simulink model "sm_tVtest_belt_IdlerArm_i2u0r3_lowerframe"  (R2026a)
settings: Solver=ode23t  StopTime=16  AbsTol=1e-3  EnableMultiTasking=on
StartFcn:
  | tic
StopFcn:
  | Elapsed_Sim_Time = toc;
  | disp(['Elapsed Sim Time = ' num2str(Elapsed_Sim_Time)]);
undefined symbols (not defined in the file or in its folder): A, L1, L2, L3, qSegSpr_seg45i2u0r3, S, sprk_pitch_rad, X, Y, Z
libraries: sm_lib x7, sm_trackV_lib_belt_contact_internal_sets x7, fl_lib x2, nesl_utility x2, sm_trackV_lib_chain_underc_elem x1, simulink x1, sm_trackV_lib_terrain_contact_s45 x1, sm_trackV_lib_belt_track_s45 x1, sm_trackV_lib_belt_underc_idlerArm_i2u0l3 x1
Description:
  | Belt with Undercarriage, Ground Contact Point Cloud
  | Copyright 2024-2026 The MathWorks, Inc.
settings Model: Creator=smiller  LastModifiedBy=smiller
settings DataIOCC: SignalLoggingName=logsout_sm_tVtest_belt_IdlerArm_i2u0r3_lowerframe
settings DebuggingCC: SubsystemReferenceDiagnosticForUnitTest=warning
settings SimscapeCC: SimscapeNominalValues="[{\"value\":\"1\",\"unit\":\"A\"},{\"value\":\"1\",\"unit\":\"bar\"},{\"value\":\"1\",\"unit\":\"cm^2\"},{\"value\":\"1\",\"unit\":\"cm^3/s\"},{\"value\":\"1\",\"unit\":\"kJ/kg\"},{\"value\":\"1\",\"unit\":\"kW\"},{\"value\":\"1\",\"unit\":\"l\"},{\"value\":\"1\",\"unit\":\"N\"},{\"value\":\"1\",\"unit\":\"N*m\"},{\"value\":\"1\",\"unit\":\"V\"}]"  SimscapeLogSimulationStatistics=on  SimscapeLogName=simlog_sm_tVtest_belt_IdlerArm_i2u0r3_lowerframe  SimscapeLogLimitData=off
settings DiagnosticsConfigSet: SimMechanicsUnconnectedFramePorts=none
settings ExplorerConfigSet: InternalSimMechanicsExplorerSettings="<ExplorerConfiguration><canonicalview>default</canonicalview><AnimationSetting><BasePlaybackSpeed>1.0</BasePlaybackSpeed><PlaybackSpeedFactor>1.0</PlaybackSpeedFactor></AnimationSetting><TilePanel><TileInfo><Tiles Columns=\"1\" Count=\"1\" Rows=\"1\"><Column Weight=\"1\"/><Row Weight=\"1\"/><Tile Height=\"1\" Width=\"1\" X=\"0\" Y=\"0\"/></Tiles></TileInfo><SceneInfo><SceneViewer><BGColor><R>1</R><G>1</G><B>1</B></BGColor><Camera><DoPerspective>off</DoPerspective><Position><X>0.47068243127928272</X><Y>-1.75489189973030935</Y><Z>1.25342844941222076</Z></Position><Center><X>-0.0540333939973325975</X><Y>-0.199725656684764663</Y><Z>0.955761903192511197</Z></Center><Up><X>-0.029483751236791006</X><Y>0.178305307946765135</Y><Z>0.983533388132307618</Z></Up><ViewLimDist>1</ViewLimDist><YLim>1.28706962276995207</YLim><XLim>2.19495206711441337</XLim></Camera></SceneViewer></SceneInfo></TilePanel><MechEditorPanel><Cameras/><GfxPanelCameraMap/><VideoCreator><PlaybackSpeedRatio>1.0</PlaybackSpeedRatio><FrameRate>30</FrameRate><VideoFormat>Motion JPEG AVI</VideoFormat><FrameSize>auto</FrameSize></VideoCreator></MechEditorPanel></ExplorerConfiguration>"

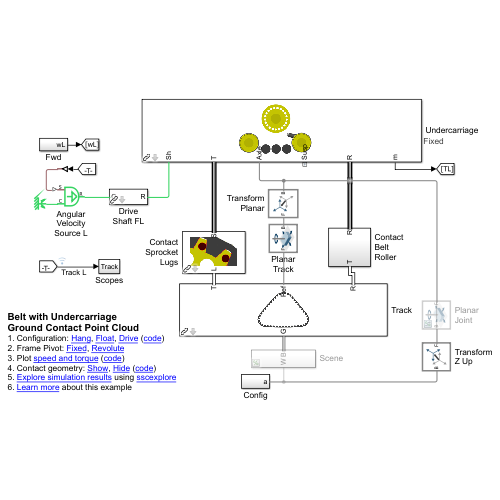
[thumbnail: Simulink's stored preview of the top-level diagram]
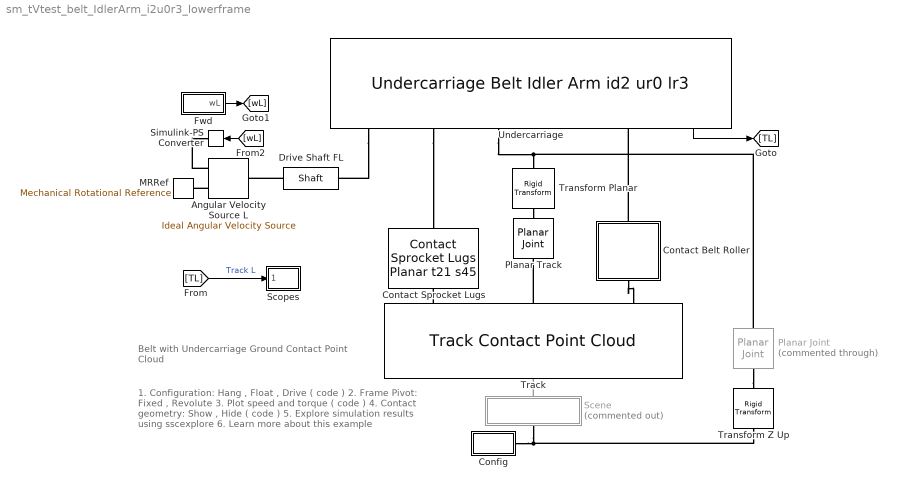
== system sm_tVtest_belt_IdlerArm_i2u0r3_lowerframe ==
  note: Belt with Undercarriage
      | Ground Contact Point Cloud
  note: 1. Configuration: Hang , Float , Drive ( code )
      | 2. Frame Pivot: Fixed , Revolute
      | 3. Plot speed and torque ( code )
      | 4. Contact geometry: Show , Hide ( code )
      | 5. Explore simulation results using sscexplore
      | 6. Learn more about this example
  Angular Velocity Source L : fl_lib/Mechanical/Mechanical Sources/Ideal Angular Velocity Source
  Config : Subsystem
  Contact Belt Roller : Subsystem
  Contact Sprocket Lugs : sm_trackV_lib_belt_contact_internal_sets/Contact Sprocket Lugs Planar t21 s45  K_SprocketLug=Trac.Contact.SprocketLug.K  B_SprocketLug=Trac.Contact.SprocketLug.B  TW_SprocketLug=Trac.Contact.SprocketLug.TW
  Drive Shaft FL : sm_trackV_lib_chain_underc_elem/Shaft  k_shaft=Excv.Drive.Shaft.k  b_shaft=Excv.Drive.Shaft.b
  Fwd : Subsystem  VariantControl=Fwd
  MRRef : fl_lib/Mechanical/Rotational Elements/Mechanical Rotational Reference
  Planar Joint : sm_lib/Joints/Planar Joint  Commented=through  JointMode=Normal  CompositeWrenchDir=FollowerOnBase  CompositeWrenchFrame=BaseFrame  SenseConstraintForce=off  SenseConstraintTorque=off  SenseTotalForce=off  SenseTotalTorque=off  PxPositionTargetSpecify=off  PxPositionTargetPriority=High  PxPositionTargetValue=0  PxPositionTargetValueUnits=m  PxVelocityTargetSpecify=off  PxVelocityTargetPriority=High  PxVelocityTargetValue=0  PxVelocityTargetValueUnits=m/s  PxEquilibriumPosition=0  PxEquilibriumPositionUnits=m  PxSpringStiffness=0  PxSpringStiffnessUnits=N/m  PxDampingCoefficient=0  PxDampingCoefficientUnits=N/(m/s)  PxLowerLimitSpecify=off  PxLowerLimitBound=-1  PxLowerLimitBoundUnits=m  PxLowerLimitStiffness=1e6  PxLowerLimitStiffnessUnits=N/m  PxLowerLimitDamping=1e3  PxLowerLimitDampingUnits=N/(m/s)  PxLowerLimitTransitionRegionWidth=1e-4  PxLowerLimitTransitionRegionWidthUnits=m  PxUpperLimitSpecify=off  PxUpperLimitBound=1  PxUpperLimitBoundUnits=m  PxUpperLimitStiffness=1e6  PxUpperLimitStiffnessUnits=N/m  PxUpperLimitDamping=1e3  PxUpperLimitDampingUnits=N/(m/s)  PxUpperLimitTransitionRegionWidth=1e-4  PxUpperLimitTransitionRegionWidthUnits=m  PxTorqueActuationMode=NoTorque  PxMotionActuationMode=ComputedMotion  PxSensePosition=off  PxSenseVelocity=off  PxSenseAcceleration=off  PxSenseTorqueForce=off  PxSenseLowerLimitTorqueForce=off  PxSenseUpperLimitTorqueForce=off  PyPositionTargetSpecify=off  PyPositionTargetPriority=High  PyPositionTargetValue=0  PyPositionTargetValueUnits=m  PyVelocityTargetSpecify=off  PyVelocityTargetPriority=High  PyVelocityTargetValue=0  PyVelocityTargetValueUnits=m/s  PyEquilibriumPosition=0  PyEquilibriumPositionUnits=m  PySpringStiffness=0  PySpringStiffnessUnits=N/m  PyDampingCoefficient=0  PyDampingCoefficientUnits=N/(m/s)  PyLowerLimitSpecify=off  PyLowerLimitBound=-1  PyLowerLimitBoundUnits=m  PyLowerLimitStiffness=1e6  PyLowerLimitStiffnessUnits=N/m  PyLowerLimitDamping=1e3  PyLowerLimitDampingUnits=N/(m/s)  PyLowerLimitTransitionRegionWidth=1e-4  PyLowerLimitTransitionRegionWidthUnits=m  PyUpperLimitSpecify=off  PyUpperLimitBound=1  PyUpperLimitBoundUnits=m  PyUpperLimitStiffness=1e6  PyUpperLimitStiffnessUnits=N/m  PyUpperLimitDamping=1e3  PyUpperLimitDampingUnits=N/(m/s)  PyUpperLimitTransitionRegionWidth=1e-4  PyUpperLimitTransitionRegionWidthUnits=m  PyTorqueActuationMode=NoTorque  PyMotionActuationMode=ComputedMotion  PySensePosition=off  PySenseVelocity=off  PySenseAcceleration=off  PySenseTorqueForce=off  PySenseLowerLimitTorqueForce=off  PySenseUpperLimitTorqueForce=off  RzPositionTargetSpecify=off  RzPositionTargetPriority=High  RzPositionTargetValue=0  RzPositionTargetValueUnits=deg  RzVelocityTargetSpecify=off  RzVelocityTargetPriority=High  RzVelocityTargetValue=0  RzVelocityTargetValueUnits=deg/s  RzEquilibriumPosition=0  RzEquilibriumPositionUnits=deg  RzSpringStiffness=0  RzSpringStiffnessUnits=N*m/deg  RzDampingCoefficient=0  RzDampingCoefficientUnits=N*m/(deg/s)  RzLowerLimitSpecify=off  RzLowerLimitBound=-90  RzLowerLimitBoundUnits=deg  RzLowerLimitStiffness=1e4  RzLowerLimitStiffnessUnits=N*m/deg  RzLowerLimitDamping=10  RzLowerLimitDampingUnits=N*m/(deg/s)  RzLowerLimitTransitionRegionWidth=0.1  RzLowerLimitTransitionRegionWidthUnits=deg  RzUpperLimitSpecify=off  RzUpperLimitBound=90  RzUpperLimitBoundUnits=deg  RzUpperLimitStiffness=1e4  RzUpperLimitStiffnessUnits=N*m/deg  RzUpperLimitDamping=10  RzUpperLimitDampingUnits=N*m/(deg/s)  RzUpperLimitTransitionRegionWidth=0.1  RzUpperLimitTransitionRegionWidthUnits=deg  RzTorqueActuationMode=NoTorque  RzMotionActuationMode=ComputedMotion  RzSensePosition=off  RzSenseVelocity=off  RzSenseAcceleration=off  RzSenseTorqueForce=off  RzSenseLowerLimitTorqueForce=off  RzSenseUpperLimitTorqueForce=off
  Planar Track : sm_lib/Joints/Planar Joint  JointMode=Normal  CompositeWrenchDir=FollowerOnBase  CompositeWrenchFrame=BaseFrame  SenseConstraintForce=off  SenseConstraintTorque=off  SenseTotalForce=off  SenseTotalTorque=off  PxPositionTargetSpecify=off  PxPositionTargetPriority=High  PxPositionTargetValue=0  PxPositionTargetValueUnits=m  PxVelocityTargetSpecify=off  PxVelocityTargetPriority=High  PxVelocityTargetValue=0  PxVelocityTargetValueUnits=m/s  PxEquilibriumPosition=0  PxEquilibriumPositionUnits=m  PxSpringStiffness=0  PxSpringStiffnessUnits=N/m  PxDampingCoefficient=0  PxDampingCoefficientUnits=N/(m/s)  PxLowerLimitSpecify=off  PxLowerLimitBound=-1  PxLowerLimitBoundUnits=m  PxLowerLimitStiffness=1e6  PxLowerLimitStiffnessUnits=N/m  PxLowerLimitDamping=1e3  PxLowerLimitDampingUnits=N/(m/s)  PxLowerLimitTransitionRegionWidth=1e-4  PxLowerLimitTransitionRegionWidthUnits=m  PxUpperLimitSpecify=off  PxUpperLimitBound=1  PxUpperLimitBoundUnits=m  PxUpperLimitStiffness=1e6  PxUpperLimitStiffnessUnits=N/m  PxUpperLimitDamping=1e3  PxUpperLimitDampingUnits=N/(m/s)  PxUpperLimitTransitionRegionWidth=1e-4  PxUpperLimitTransitionRegionWidthUnits=m  PxTorqueActuationMode=NoTorque  PxMotionActuationMode=ComputedMotion  PxSensePosition=off  PxSenseVelocity=off  PxSenseAcceleration=off  PxSenseTorqueForce=off  PxSenseLowerLimitTorqueForce=off  PxSenseUpperLimitTorqueForce=off  PyPositionTargetSpecify=off  PyPositionTargetPriority=Low  PyPositionTargetValue=-sprk_pitch_rad  PyPositionTargetValueUnits=m  PyVelocityTargetSpecify=off  PyVelocityTargetPriority=High  PyVelocityTargetValue=0  PyVelocityTargetValueUnits=m/s  PyEquilibriumPosition=0  PyEquilibriumPositionUnits=m  PySpringStiffness=0  PySpringStiffnessUnits=N/m  PyDampingCoefficient=0  PyDampingCoefficientUnits=N/(m/s)  PyLowerLimitSpecify=off  PyLowerLimitBound=-1  PyLowerLimitBoundUnits=m  PyLowerLimitStiffness=1e6  PyLowerLimitStiffnessUnits=N/m  PyLowerLimitDamping=1e3  PyLowerLimitDampingUnits=N/(m/s)  PyLowerLimitTransitionRegionWidth=1e-4  PyLowerLimitTransitionRegionWidthUnits=m  PyUpperLimitSpecify=off  PyUpperLimitBound=1  PyUpperLimitBoundUnits=m  PyUpperLimitStiffness=1e6  PyUpperLimitStiffnessUnits=N/m  PyUpperLimitDamping=1e3  PyUpperLimitDampingUnits=N/(m/s)  PyUpperLimitTransitionRegionWidth=1e-4  PyUpperLimitTransitionRegionWidthUnits=m  PyTorqueActuationMode=NoTorque  PyMotionActuationMode=ComputedMotion  PySensePosition=off  PySenseVelocity=off  PySenseAcceleration=off  PySenseTorqueForce=off  PySenseLowerLimitTorqueForce=off  PySenseUpperLimitTorqueForce=off  RzPositionTargetSpecify=on  RzPositionTargetPriority=High  RzPositionTargetValue=0  RzPositionTargetValueUnits=deg  RzVelocityTargetSpecify=off  RzVelocityTargetPriority=High  RzVelocityTargetValue=0  RzVelocityTargetValueUnits=deg/s  RzEquilibriumPosition=0  RzEquilibriumPositionUnits=deg  RzSpringStiffness=0  RzSpringStiffnessUnits=N*m/deg  RzDampingCoefficient=0  RzDampingCoefficientUnits=N*m/(deg/s)  RzLowerLimitSpecify=off  RzLowerLimitBound=-90  RzLowerLimitBoundUnits=deg  RzLowerLimitStiffness=1e4  RzLowerLimitStiffnessUnits=N*m/deg  RzLowerLimitDamping=10  RzLowerLimitDampingUnits=N*m/(deg/s)  RzLowerLimitTransitionRegionWidth=0.1  RzLowerLimitTransitionRegionWidthUnits=deg  RzUpperLimitSpecify=off  RzUpperLimitBound=90  RzUpperLimitBoundUnits=deg  RzUpperLimitStiffness=1e4  RzUpperLimitStiffnessUnits=N*m/deg  RzUpperLimitDamping=10  RzUpperLimitDampingUnits=N*m/(deg/s)  RzUpperLimitTransitionRegionWidth=0.1  RzUpperLimitTransitionRegionWidthUnits=deg  RzTorqueActuationMode=NoTorque  RzMotionActuationMode=ComputedMotion  RzSensePosition=off  RzSenseVelocity=off  RzSenseAcceleration=off  RzSenseTorqueForce=off  RzSenseLowerLimitTorqueForce=off  RzSenseUpperLimitTorqueForce=off
  Scene : Subsystem  Commented=on
  Scopes : Subsystem
  Simulink-PS Converter : nesl_utility/Simulink-PS Converter  PhysicalDomain=network_engine_domain  SubClassName=ps_input  LeftPortType=input  RightPortType=output  PseudoPeriodic=off  Frequencies=[]  NoiseDistribution=none  NoiseParameters=[]  Unit=1  AffineConversion=off  FilteringAndDerivatives=provide  SimscapeFilterOrder=1  InputFilterTimeConstant=0.001  UdotUserProvided=0
  Track : sm_trackV_lib_belt_track_s45/Track Contact Point Cloud  carc_len=Trac.Belt.l  carc_wid=Trac.Belt.w  carc_thk=Trac.Belt.pad_h  carc_mass=Trac.Belt.mass  carc_cg=Trac.Belt.cg  carc_moi=Trac.Belt.moi  carc_poi=Trac.Belt.poi  carc_clr=Trac.Belt.clr  carc_opc=Trac.Belt.opc  lug_hei=Trac.Belt.Lug.h  lug_lb=Trac.Belt.Lug.lb  lug_lt=Trac.Belt.Lug.lt  lug_w=Trac.Belt.Lug.w  lug_xc=Trac.Belt.Lug.xc  lug_clr=Trac.Belt.clr  lug_opc=Trac.Belt.opc  jointTargets=track_seg_tgts_seg45i2u0r3  trackDamping=Trac.Belt.damping  lug_line_clr=Trac.Belt.lug_contact.clr  lug_line_opc=Trac.Belt.lug_contact.opc  carc_line_clr=Trac.Belt.carcass_contact.clr  carc_line_opc=Trac.Belt.carcass_contact.opc  ptcld_belt=Trac.Belt.ground_contact.ptcld.pts  ptcld_belt_rad=Trac.Belt.ground_contact.ptcld.rad  ptcld_belt_clr=Trac.Belt.ground_contact.ptcld.clr  ptcld_belt_opc=Trac.Belt.ground_contact.ptcld.opc
  Transform Planar : sm_lib/Frames and Transforms/Rigid Transform  RotationMethod=StandardAxis  FollAlignAxisA=+X  BaseAlignAxisA=+Y  FollAlignAxisB=+Y  BaseAlignAxisB=+Z  RotationStandardAxis=+Z  RotationAngle=-qSegSpr_seg45i2u0r3/2  RotationAngleUnits=deg  RotationArbitraryAxis=[0 0 1]  RotationSequenceAxes=FollowerAxes  RotationSequence=XYX  RotationSequenceAngles=[0 0 0]  RotationSequenceAnglesUnits=deg  RotationMatrix=[1 0 0; 0 1 0; 0 0 1]  Quaternion=[1 0 0 0]  TranslationMethod=StandardAxis  TranslationCartesianOffset=[0 0 0]  TranslationCartesianOffsetUnits=m  TranslationStandardAxis=+Y  TranslationStandardOffset=-sprk_pitch_rad  TranslationStandardOffsetUnits=m  TranslationROffset=0  TranslationROffsetUnits=m  TranslationThetaOffset=0  TranslationThetaOffsetUnits=deg  TranslationZOffset=0  TranslationZOffsetUnits=m
  Transform Z Up : sm_lib/Frames and Transforms/Rigid Transform  RotationMethod=StandardAxis  FollAlignAxisA=+X  BaseAlignAxisA=+Y  FollAlignAxisB=+Y  BaseAlignAxisB=+Z  RotationStandardAxis=+X  RotationAngle=-90  RotationAngleUnits=deg  RotationArbitraryAxis=[0 0 1]  RotationSequenceAxes=FollowerAxes  RotationSequence=XYX  RotationSequenceAngles=[0 0 0]  RotationSequenceAnglesUnits=deg  RotationMatrix=[1 0 0; 0 1 0; 0 0 1]  Quaternion=[1 0 0 0]  TranslationMethod=StandardAxis  TranslationCartesianOffset=[0 0 0]  TranslationCartesianOffsetUnits=m  TranslationStandardAxis=+Z  TranslationStandardOffset=1.5  TranslationStandardOffsetUnits=m  TranslationROffset=0  TranslationROffsetUnits=m  TranslationThetaOffset=0  TranslationThetaOffsetUnits=deg  TranslationZOffset=0  TranslationZOffsetUnits=m
  Undercarriage : sm_trackV_lib_belt_underc_idlerArm_i2u0l3/Undercarriage Belt Idler Arm id2 ur0 lr3  popup_leftOrRight=Right  sprk_rad_roll=Trac.Sprocket.Roller.rad  sprk_wid_roll=Trac.Sprocket.Roller.wid  sprk_clr=Trac.Sprocket.Roller.clr  sprk_opc=Trac.Sprocket.Roller.opc  sprk_rim_ir=Trac.Sprocket.Rim.rad_inner  sprk_rim_thk=Trac.Sprocket.Rim.thk  sprk_rim_spoke_xc=Trac.Sprocket.Rim.spoke_xc  sprk_rad_pitch=Trac.Sprocket.Spoke.pitch_rad  sprk_spoke_rad=Trac.Sprocket.Spoke.rad  sprk_spoke_len=Trac.Sprocket.Spoke.len  sprk_spoke_num=Trac.Sprocket.nSpokes  sprk_contgeo_roller_clr=Trac.Sprocket.roller_contact.clr  sprk_contgeo_roller_opc=Trac.Sprocket.roller_contact.opc  sprk_contgeo_spoke_clr=Trac.Sprocket.spoke_contact.clr  sprk_contgeo_spoke_opc=Trac.Sprocket.spoke_contact.opc  idlerR_rad=Trac.IdlerR.rad  idlerF_rad=Trac.IdlerF.rad  idlerR_len=Trac.IdlerR.len  idlerF_len=Trac.IdlerF.len  idlerR_rho=Trac.IdlerR.rho  idlerF_rho=Trac.IdlerF.rho  idlerR_wheel_clr=Trac.IdlerR.Wheel.clr  idlerF_wheel_clr=Trac.IdlerF.Wheel.clr  idlerR_rim_rad=Trac.IdlerR.Rim.rad  idlerF_rim_rad=Trac.IdlerF.Rim.rad  idlerR_rim_hub_rad=Trac.IdlerR.Rim.hub_rad  idlerF_rim_hub_rad=Trac.IdlerF.Rim.hub_rad  idlerR_rim_xc=Trac.IdlerR.Rim.rim_xc  idlerF_rim_xc=Trac.IdlerF.Rim.rim_xc  idlerR_clr=Trac.IdlerR.clr  idlerF_clr=Trac.IdlerF.clr  idlerR_opc=Trac.IdlerR.opc  idlerF_opc=Trac.IdlerF.opc  idlerR_axle_rad=Trac.IdlerR.Axle.rad  idlerF_axle_rad=Trac.IdlerF.Axle.rad  idlerR_axle_len=Trac.IdlerR.Axle.len  idlerF_axle_len=Trac.IdlerF.Axle.len  idlerR_axle_rho=Trac.IdlerR.Axle.rho  idlerF_axle_rho=Trac.IdlerF.Axle.rho  idlerR_axle_clr=Trac.IdlerR.Axle.clr  idlerF_axle_clr=Trac.IdlerF.Axle.clr  idlerR_axle_opc=Trac.IdlerR.Axle.opc  idlerF_axle_opc=Trac.IdlerF.Axle.opc  idlerR_contgeo_clr=Trac.IdlerR.belt_contact.clr  idlerF_contgeo_clr=Trac.IdlerF.belt_contact.clr  idlerR_contgeo_opc=Trac.IdlerR.belt_contact.opc  idlerF_contgeo_opc=Trac.IdlerF.belt_contact.opc  arm_idlerc=Trac.IdlerArm.Pivot_to_Idler  arm_tens_x=Trac.IdlerArm.Pivot_to_TensionerX  arm_tens_y=Trac.IdlerArm.Pivot_to_TensionerY  arm_wid=Trac.IdlerArm.wid  arm_thk=Trac.IdlerArm.thk  arm_rho=Trac.IdlerArm.rho  arm_clr=Trac.IdlerArm.clr  arm_opc=Trac.IdlerArm.opc  roller_lower_len=Trac.Roller.Lower.len  roller_lower_rad=Trac.Roller.Lower.rad  roller_lower_rho=Trac.Roller.Lower.rho  roller_lower_clr=Trac.Roller.Lower.clr  roller_lower_opc=Trac.Roller.Lower.opc  roller_lower_rim_thk=Trac.Roller.Lower.rim_thk  roller_lower_rim_len=Trac.Roller.Lower.rim_len  roller_lower_axle_len=Trac.Roller.Lower.Axle.len  roller_lower_axle_rad=Trac.Roller.Lower.Axle.rad  roller_lower_axle_rho=Trac.Roller.Lower.Axle.rho  roller_lower_axle_clr=Trac.Roller.Lower.Axle.clr  roller_lower_axle_opc=Trac.Roller.Lower.Axle.opc  roller_lower_contgeo_clr=Trac.Roller.Lower.belt_contact.clr  roller_lower_contgeo_opc=Trac.Roller.Lower.belt_contact.opc  tensioner_cyl_len=Trac.IdlerF.Tensioner.cyl.len  tensioner_cyl_rad=Trac.IdlerF.Tensioner.cyl.rad  tensioner_cyl_rho=Trac.IdlerF.Tensioner.cyl.rho  tensioner_cyl_clr=Trac.IdlerF.Tensioner.cyl.clr  tensioner_cyl_opc=Trac.IdlerF.Tensioner.cyl.opc  tensioner_pist_len=Trac.IdlerF.Tensioner.piston.len  tensioner_pist_rad=Trac.IdlerF.Tensioner.piston.rad  tensioner_pist_rho=Trac.IdlerF.Tensioner.piston.rho  tensioner_pist_clr=Trac.IdlerF.Tensioner.piston.clr  tensioner_pist_opc=Trac.IdlerF.Tensioner.piston.opc  tensioner_br_len=Trac.IdlerF.Tensioner.bracket.len  tensioner_br_width=Trac.IdlerF.Tensioner.bracket.wid  tensioner_br_height=Trac.IdlerF.Tensioner.bracket.height  tensioner_br_thk=Trac.IdlerF.Tensioner.bracket.thk  tensioner_br_rho=Trac.IdlerF.Tensioner.bracket.rho  tensioner_br_clr=Trac.IdlerF.Tensioner.bracket.clr  tensioner_br_opc=Trac.IdlerF.Tensioner.bracket.opc  tensioner_eqpos=Trac.IdlerF.Tensioner.xeq  tensioner_x0=Trac.IdlerF.Tensioner.x0  tensioner_k=Trac.IdlerF.Tensioner.K  tensioner_b=Trac.IdlerF.Tensioner.B  popup_trackFrame=Fixed  roller_lower_x=Trac.Frame.SprkOffLon.Lower  axle_x=Trac.Frame.SprkOffLon.Axle  idlerFix_x=Trac.Frame.SprkOffLon.IdlerR  frame_pivot_x=Trac.Frame.SprkOffLon.PivotFra  tensionC_x=Trac.Frame.SprkOffLon.TensionC  idlerArm_x=Trac.Frame.SprkOffLon.IdlerArm  roller_lower_y=Trac.Frame.SprkOffVer.Lower  axle_y=Trac.Frame.SprkOffVer.Axle  idlerArm_y=Trac.Frame.SprkOffVer.IdlerArm  idlerFix_y=Trac.Frame.SprkOffVer.IdlerR  frame_pivot_y=Trac.Frame.SprkOffVer.PivotFra  tensionC_y=Trac.Frame.SprkOffVer.TensionC  frame_cg_offset=Trac.Frame.TrackFrame.CG  frame_mass=Trac.Frame.TrackFrame.Mass  frame_moi=Trac.Frame.TrackFrame.MOI  frame_poi=Trac.Frame.TrackFrame.POI  frame_roller_cg_offset=Trac.Frame.SprkFrame.CG  frame_roller_mass=Trac.Frame.SprkFrame.Mass  frame_roller_moi=Trac.Frame.SprkFrame.MOI  frame_roller_poi=Trac.Frame.SprkFrame.POI  roller_frame_pivot_range=Trac.Frame.PivotFra.Range  roller_frame_pivot_k=Trac.Frame.PivotFra.LimitK  roller_frame_pivot_b=Trac.Frame.PivotFra.LimitB  roller_frame_pivot_tw=Trac.Frame.PivotFra.LimitTW  frame_susp_offset=Trac.Frame.SuspOffset  popup_sense_roller=Actuator Torque
      settings: AttributesFormatString=%<popup_trackFrame>
  wires:
  Fwd/1(wL) -> [wL]
  [wL] -> Simulink-PS Converter/1
  Undercarriage/1 -> [TL]
  [TL] -> Scopes/1(Track)  "Track L"
  connections:
  Transform Planar/RConn1 -- Planar Track/LConn1
  Angular Velocity Source L/RConn2 -- MRRef/LConn1
  Drive Shaft FL/LConn1 -- Angular Velocity Source L/LConn1
  Undercarriage/RConn5 -- Drive Shaft FL/RConn1
  Contact Belt Roller/LConn1 -- Track/RConn3
  Contact Belt Roller/RConn1 -- Undercarriage/RConn1
  Track/RConn2 -- Planar Track/RConn1
  Track/RConn1 -- Contact Sprocket Lugs/RConn1
  Undercarriage/RConn4 -- Contact Sprocket Lugs/LConn1
  Planar Joint/RConn1 -- Transform Planar/LConn1 -- Undercarriage/RConn3
  Planar Joint/LConn1 -- Transform Z Up/RConn1
  Angular Velocity Source L/RConn1 -- Simulink-PS Converter/RConn1
  Transform Z Up/LConn1 -- Config/RConn1 -- Scene/LConn1
  Scene/RConn1 -- Track/LConn1

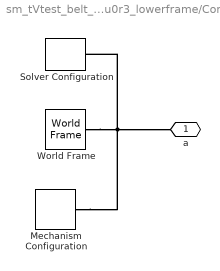
== system sm_tVtest_belt_IdlerArm_i2u0r3_lowerframe/Config ==
  Mechanism Configuration : sm_lib/Utilities/Mechanism Configuration  UniformGravity=Constant  GravityVector=[0 0 -9.80665]  GravityVectorUnits=m/s^2  LinearizationDelta=0.001  JointModeTransitionNonlinearIterations=2
  Solver Configuration : nesl_utility/Solver Configuration  PhysicalDomain=network_engine_domain  SubClassName=solver  LeftPortType=input  RightPortType=generic  Tones=[]  Harmonics=[]  SimulateNoise=off  Profile=off  UseLocalSampling=off  EnableSwitchedLinearOptims=on  FrequencyDomain=off  UseCCode=off  RelTol=0.001  AbsTol=1e-06  MinStep=1e-09  ToWorkspace=off  RevertToSquareIcSolve=off  NumHomotopyIterations=100  PhasorMode=off  PhasorModeNumHarmonics=1  ConsistencySolver=NEWTON_XTOL_AFTER_FTOL  CanonicalOrdering=UNORDERED  OptimizeIntermediates=UNOPTIMIZED  IndexReductionMethod=DerivativeReplacement  DoDC=off  ResidualTolerance=1e-09  ConsistencyTolSource=GLOBAL  ConsistencyAbsTol=0.001  ConsistencyRelTol=0.001  ConsistencyTolFactor=0.001  UseLocalSolver=off  LocalSolverChoice=NE_BACKWARD_EULER_ADVANCER  ResolveIndetEquations=on  FunctionEvalNumThread=1  LocalSolverSampleTime=0.001  DoFixedCost=off  MaxNonlinIter=3  MaxModeIter=2  ComputeImpulses=off  ImpulseIterations=2  LinearAlgebra=Sparse  LinearAlgebraNumThread=0  EquationFormulation=NE_TIME_EF  DelaysMemoryBudget=1024  AutomaticFiltering=on  FilteringTimeConstant=0.001  PartitionStorageMethod=AS_NEEDED  PartitionMemoryBudget=1024  PartitionMethod=FAST  MultibodyUseLocalSolver=off  MultibodyLocalSolverChoice=ODE1  MultibodyLocalSolverSampleTime=0.001
  World Frame : sm_lib/Frames and Transforms/World Frame
  a : PMIOPort  Side=Right
  connections:
  World Frame/RConn1 -- a/RConn1 -- Solver Configuration/RConn1 -- Mechanism Configuration/RConn1

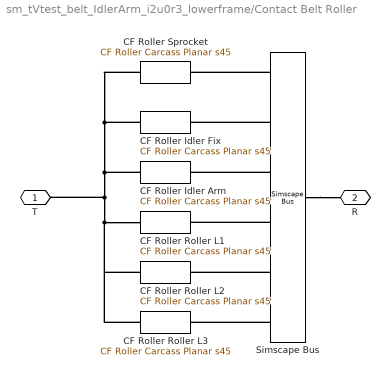
== system sm_tVtest_belt_IdlerArm_i2u0r3_lowerframe/Contact Belt Roller ==
  CF Roller Idler Arm : sm_trackV_lib_belt_contact_internal_sets/CF Roller Carcass Planar s45  K_Roller=Trac.Contact.IdlerF.K  B_Roller=Trac.Contact.IdlerF.B  TW_Roller=Trac.Contact.IdlerF.TW
  CF Roller Idler Fix : sm_trackV_lib_belt_contact_internal_sets/CF Roller Carcass Planar s45  K_Roller=Trac.Contact.IdlerR.K  B_Roller=Trac.Contact.IdlerR.B  TW_Roller=Trac.Contact.IdlerR.TW
  CF Roller Roller L1 : sm_trackV_lib_belt_contact_internal_sets/CF Roller Carcass Planar s45  K_Roller=Trac.Contact.Roller.K  B_Roller=Trac.Contact.Roller.B  TW_Roller=Trac.Contact.Roller.TW
  CF Roller Roller L2 : sm_trackV_lib_belt_contact_internal_sets/CF Roller Carcass Planar s45  K_Roller=Trac.Contact.Roller.K  B_Roller=Trac.Contact.Roller.B  TW_Roller=Trac.Contact.Roller.TW
  CF Roller Roller L3 : sm_trackV_lib_belt_contact_internal_sets/CF Roller Carcass Planar s45  K_Roller=Trac.Contact.Roller.K  B_Roller=Trac.Contact.Roller.B  TW_Roller=Trac.Contact.Roller.TW
  CF Roller Sprocket : sm_trackV_lib_belt_contact_internal_sets/CF Roller Carcass Planar s45  K_Roller=Trac.Contact.SprocketRoller.K  B_Roller=Trac.Contact.SprocketRoller.B  TW_Roller=Trac.Contact.SprocketRoller.TW
  Simscape Bus : SimscapeBus  HierarchyStrings=S;X;A;L1;L2;L3
  T : PMIOPort  Side=Left
  R : PMIOPort  Port=2  Side=Right
  connections:
  Simscape Bus/LConn3 -- CF Roller Idler Arm/LConn1
  Simscape Bus/LConn4 -- CF Roller Roller L1/LConn1
  CF Roller Sprocket/RConn1 -- CF Roller Idler Fix/RConn1 -- CF Roller Idler Arm/RConn1 -- T/RConn1 -- CF Roller Roller L2/RConn1 -- CF Roller Roller L3/RConn1 -- CF Roller Roller L1/RConn1
  Simscape Bus/LConn2 -- CF Roller Idler Fix/LConn1
  Simscape Bus/RConn1 -- R/RConn1
  Simscape Bus/LConn5 -- CF Roller Roller L2/LConn1
  Simscape Bus/LConn1 -- CF Roller Sprocket/LConn1
  Simscape Bus/LConn6 -- CF Roller Roller L3/LConn1

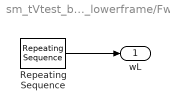
== system sm_tVtest_belt_IdlerArm_i2u0r3_lowerframe/Fwd ==
  Repeating Sequence : simulink/Sources/Repeating Sequence  rep_seq_t=[0 2 2.01 40]  rep_seq_y=[0 0 3 3]*0.744
  wL : Outport
  wires:
  Repeating Sequence/1 -> wL/1

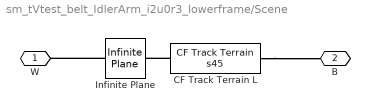
== system sm_tVtest_belt_IdlerArm_i2u0r3_lowerframe/Scene ==
  CF Track Terrain L : sm_trackV_lib_terrain_contact_s45/CF Track Terrain s45  K_Road=Scene.Contact.Terrain.K  B_Road=Scene.Contact.Terrain.B  TW_Road=Scene.Contact.Terrain.TW  F_dyn_Road=Scene.Contact.Terrain.mud  F_stat_Road=Scene.Contact.Terrain.mus  CV_Road=Scene.Contact.Terrain.CV
  Infinite Plane : sm_lib/Curves and Surfaces/Infinite Plane  GraphicType=Rectangle  GraphicPlaneWidth=4  GraphicPlaneWidthUnits=m  GraphicPlaneHeight=2  GraphicPlaneHeightUnits=m  GraphicVisPropType=SimpleVisualProperties  GraphicDiffuseColor=[0.5 0.5 0.5]  GraphicOpacity=0.25  GraphicSpecularColor=[0.5 0.5 0.5 1.0]  GraphicAmbientColor=[0.15 0.15 0.15 1.0]  GraphicEmissiveColor=[0.0 0.0 0.0 1.0]  GraphicShininess=75
  W : PMIOPort  Side=Left
  B : PMIOPort  Port=2  Side=Right
  connections:
  Infinite Plane/LConn1 -- W/RConn1
  CF Track Terrain L/LConn1 -- Infinite Plane/RConn1
  CF Track Terrain L/RConn1 -- B/RConn1

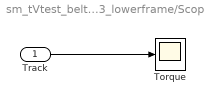
== system sm_tVtest_belt_IdlerArm_i2u0r3_lowerframe/Scopes ==
  Track : Inport
  Torque : Scope
  wires:
  Track/1 -> Torque/1
